simulink model "MassXYSimulation"  (R2013b)
settings: Solver=ode45  StartTime=0.0  StopTime=85.71  RelTol=1e-3
libraries: simulink x1
settings Model: Creator=DEL  LastModifiedBy=DEL

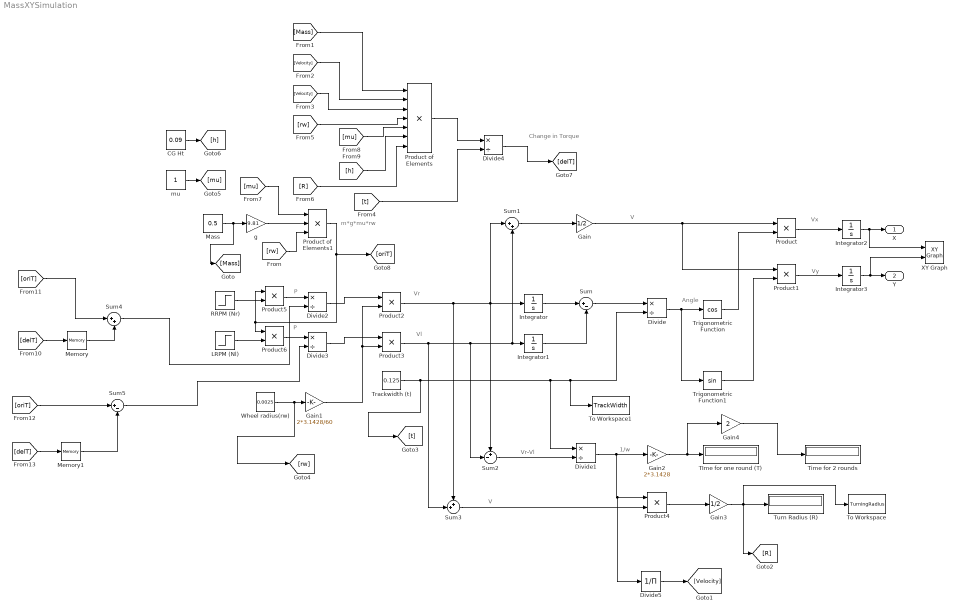
== system MassXYSimulation ==
  note: P
  note: P
  note: Change in Torque
  note: m*g*mu*rw
  note: Vr-Vl
  note: V
  note: 1/w
  note: Vl
  note: Vr
  note: Vy
  note: Vx
  note: Angle
  note: V
  CG Ht : Constant  Value=0.09
  Divide{,1..4} (5 alike) : Product  Inputs=*/
  Divide5 : Product  Inputs=/
  Gain : Gain  Gain=1/2
  Gain1 : Gain  Gain=2*3.1428/60
  Gain2 : Gain  Gain=2*3.1428
  Gain3 : Gain  Gain=1/2
  Gain4 : Gain  Gain=2
  Integrator{,1..3} (4 alike) : Integrator
  LRPM (Nl) : Step  Time=0  Before=230  After=230  SampleTime=0
  "Mass " : Constant  Value=0.5
  Memory : Memory
  Memory1 : Memory
  Product{,1..6} (7 alike) : Product
  Product of Elements : Product  Inputs=*******
  Product of Elements1 : Product  Inputs=***
  RRPM (Nr) : Step  Time=0  Before=300  After=300  SampleTime=0
  Sum : Sum  Inputs=|+-
  Sum1 : Sum  Inputs=|++
  Sum2 : Sum  Inputs=+-|
  Sum3 : Sum  Inputs=++|
  Sum4 : Sum  Inputs=|++
  Sum5 : Sum  Inputs=|+-
  TIme for one round (T) : Display
  Time for 2 rounds : Display
  To Workspace : ToWorkspace  VariableName=TurningRadius  SampleTime=-1
  To Workspace1 : ToWorkspace  VariableName=TrackWidth  SampleTime=-1
  Trackwidth (t) : Constant  Value=0.125
  Trigonometric Function : Trigonometry  Operator=cos
  Trigonometric Function1 : Trigonometry
  Turn Radius (R) : Display
  Wheel radius(rw) : Constant  Value=0.0025
  XY Graph : simulink/Sinks/XY Graph  xmin=-1.5  xmax=1.5  ymin=-1.5  ymax=1.5  st=-1
  "g " : Gain  Gain=9.81
  "mu " : Constant
  X : Outport
  Y : Outport  Port=2
  wires:
  Product3/1 -> Sum3/2, Sum2/2, Sum1/2, Integrator1/1
  Integrator/1 -> Sum/1
  Integrator1/1 -> Sum/2
  Sum/1 -> Divide/1
  Trackwidth (t)/1 -> [t], To Workspace1/1, Divide/2, Divide1/1
  Sum1/1 -> Gain/1
  Divide/1 -> Trigonometric Function/1, Trigonometric Function1/1
  Gain/1 -> Product/1, Product1/1
  Trigonometric Function/1 -> Product/2
  Trigonometric Function1/1 -> Product1/2
  Product/1 -> Integrator2/1
  Product1/1 -> Integrator3/1
  Integrator2/1 -> XY Graph/1, X/1
  Integrator3/1 -> XY Graph/2, Y/1
  Gain1/1 -> Product2/2, Product3/2
  Wheel radius(rw)/1 -> [rw], Gain1/1
  Gain2/1 -> Gain4/1, TIme for one round (T)/1
  Divide1/1 -> Divide5/1, Product4/1, Gain2/1
  Product2/1 -> Sum3/1, Integrator/1, Sum2/1, Sum1/1
  Sum2/1 -> Divide1/2
  Sum3/1 -> Product4/2
  Product4/1 -> Gain3/1
  Gain3/1 -> [R], To Workspace/1, Turn Radius (R)/1
  Gain4/1 -> Time for 2 rounds/1
  "Mass "/1 -> [Mass], "g "/1
  RRPM (Nr)/1 -> Product5/2
  LRPM (Nl)/1 -> Product6/2
  Product6/1 -> Divide3/1
  Product5/1 -> Divide2/1
  Divide2/1 -> Product2/1
  Divide3/1 -> Product3/1
  "g "/1 -> Product of Elements1/2
  Product of Elements1/1 -> Product5/1, Product6/1, [oriT]
  [rw] -> Product of Elements1/3
  Product of Elements/1 -> Divide4/1
  [Mass] -> Product of Elements/1
  [Velocity] -> Product of Elements/2
  [Velocity] -> Product of Elements/3
  [rw] -> Product of Elements/4
  CG Ht/1 -> [h]
  "mu "/1 -> [mu]
  [mu] -> Product of Elements1/1
  [mu] -> Product of Elements/5
  [h] -> Product of Elements/6
  Divide4/1 -> [delT]
  Sum4/1 -> Divide2/2
  Sum5/1 -> Divide3/2
  [oriT] -> Sum4/1
  [delT] -> Memory/1
  [oriT] -> Sum5/1
  [delT] -> Memory1/1
  Divide5/1 -> [Velocity]
  [t] -> Divide4/2
  [R] -> Product of Elements/7
  Memory1/1 -> Sum5/2
  Memory/1 -> Sum4/2
